simulink model "decoupling_simulation"  (R2018b)
settings: Solver=VariableStepAuto  StartTime=0.0  StopTime=3000  RelTol=1e-3  EnableMultiTasking=on
libraries: simulink x3
settings Model: Creator=38128  LastModifiedBy=99346
settings DataIOCC: LimitDataPoints=on  SaveFormat=Array
settings OptimizationCC: LifeSpan=inf
settings DebuggingCC: SolverPrmCheckMsg=warning  SFUnexpectedBacktrackingDiag=warning  SFNoUnconditionalDefaultTransitionDiag=warning  SFExecutionAtInitializationDiag=none
settings HardwareCC: ProdBitPerPointer=32  ProdBitPerSizeT=32  ProdBitPerPtrDiffT=32  ProdLargestAtomicFloat=None  ProdIntDivRoundTo=Undefined  ProdEndianess=Unspecified  ProdWordSize=32  ProdHWDeviceType=32-bit Generic
settings ModelReferenceCC: PropagateSignalLabelsOutOfModel=off
settings SFSimCC: SimUseLocalCustomCode=off
settings RTWCC: RTWUseLocalCustomCode=off
settings CodeAppCC: StateflowObjectComments=on
settings GRTTargetCC: TargetLangStandard=C89/C90 (ANSI)  GeneratePreprocessorConditionals=Disable all
settings ConfigComp: CovMetricSettings=dw  CovHtmlReporting=on  CovSaveCumulativeToWorkspaceVar=on  CovSaveSingleToWorkspaceVar=on  CovExternalEMLEnable=off  CovSFcnEnable=off

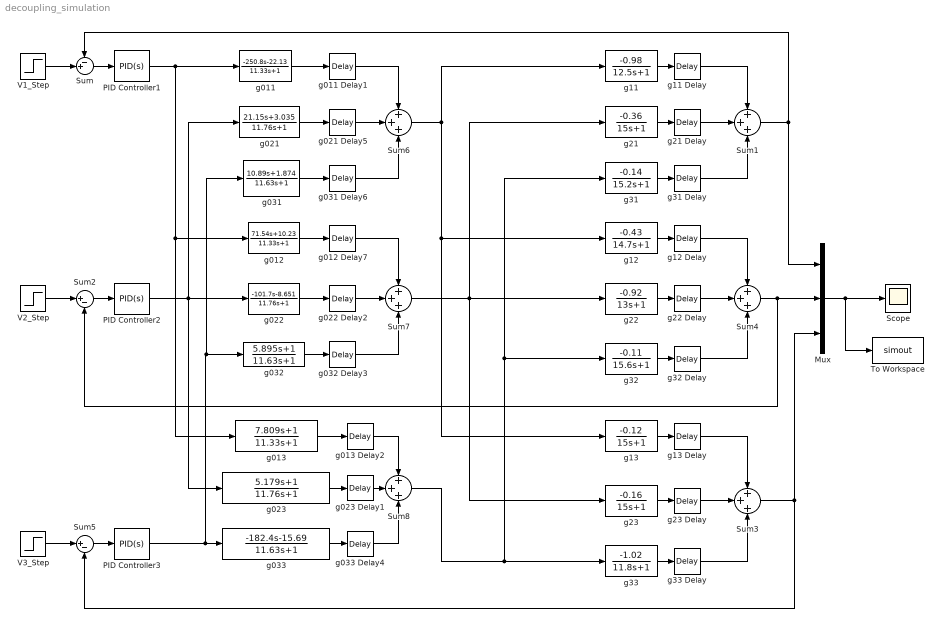
== system decoupling_simulation ==
  Mux : Mux  Inputs=3
  PID Controller1 : simulink/Continuous/PID Controller  Controller=PID  Form=Parallel  TimeDomain=Continuous-time  SampleTime=1  IntegratorMethod=Forward Euler  FilterMethod=Forward Euler  ControllerParametersSource=internal  P=0.0202  I=0.0018  D=0  UseFilter=on  N=100  TunerSelectOption=Transfer Function Based (PID Tuner App)  InitialConditionSource=internal  InitialConditionForIntegrator=0  InitialConditionForFilter=0  DifferentiatorICPrevScaledInput=0  ExternalReset=none  TrackingMode=off  Kt=1  LimitOutput=off  UpperSaturationLimit=inf  LowerSaturationLimit=-inf  LinearizeAsGain=on  AntiWindupMode=none  Kb=1  POutMin=[]  POutMax=[]  IOutMin=[]  IOutMax=[]  DOutMin=[]  DOutMax=[]  NOutMin=[]  NOutMax=[]  SumOutMin=[]  SumOutMax=[]  SaturationOutMin=[]  SaturationOutMax=[]  PParamMin=[]  PParamMax=[]  IParamMin=[]  IParamMax=[]  DParamMin=[]  DParamMax=[]  NParamMin=[]  NParamMax=[]  KbParamMin=[]  KbParamMax=[]  KtParamMin=[]  KtParamMax=[]  KbOutMin=[]  KbOutMax=[]  KtOutMin=[]  KtOutMax=[]  IntegratorOutMin=[]  IntegratorOutMax=[]  FilterOutMin=[]  FilterOutMax=[]  SumI1OutMin=[]  SumI1OutMax=[]  SumI2OutMin=[]  SumI2OutMax=[]  SumI3OutMin=[]  SumI3OutMax=[]  SumI4OutMin=[]  SumI4OutMax=[]  SumDOutMin=[]  SumDOutMax=[]  DifferentiatorOutMin=[]  DifferentiatorOutMax=[]  FilterDiffOutCoefMin=[]  FilterDiffOutCoefMax=[]  ReciprocalOutMin=[]  ReciprocalOutMax=[]  SumDenOutMin=[]  SumDenOutMax=[]  SumNumOutMin=[]  SumNumOutMax=[]  DivideOutMin=[]  DivideOutMax=[]  IntegratorContinuousStateAttributes=''  IntegratorStateMustResolveToSignalObject=off  IntegratorRTWStateStorageClass=Auto  FilterContinuousStateAttributes=''  FilterStateMustResolveToSignalObject=off  FilterRTWStateStorageClass=Auto  ParallelPVariant=InternalParameters  IdealPVariant=Disabled  IVariant=InternalParameters  DVariant=InternalParameters  IntegratorVariant=Continuous  SatVariant=Disabled  AWVariant=Passthrough  PCopyVariant=Disabled  TRVariant=Disabled  FdbkBlocksVariant=Forward  IdealPFdbkVariant=Disabled  SatFdbkVariant=Disabled  DerivativeFilterVariant=ContFilter  NVariant=InternalParameters  NCopyVariant=Disabled  FilterICVariant=InternalICsFilter  IntegratorICVariant=InternalICs  ExternalResetVariant=Disabled  TRSumVariant=Passthrough  SumFdbkVariant=Disabled  SumVariant=Sum_PID
  PID Controller2 : simulink/Continuous/PID Controller  Controller=PID  Form=Parallel  TimeDomain=Continuous-time  SampleTime=1  IntegratorMethod=Forward Euler  FilterMethod=Forward Euler  ControllerParametersSource=internal  P=0.0650  I=0.0055  D=0  UseFilter=on  N=100  TunerSelectOption=Transfer Function Based (PID Tuner App)  InitialConditionSource=internal  InitialConditionForIntegrator=0  InitialConditionForFilter=0  DifferentiatorICPrevScaledInput=0  ExternalReset=none  TrackingMode=off  Kt=1  LimitOutput=off  UpperSaturationLimit=inf  LowerSaturationLimit=-inf  LinearizeAsGain=on  AntiWindupMode=none  Kb=1  POutMin=[]  POutMax=[]  IOutMin=[]  IOutMax=[]  DOutMin=[]  DOutMax=[]  NOutMin=[]  NOutMax=[]  SumOutMin=[]  SumOutMax=[]  SaturationOutMin=[]  SaturationOutMax=[]  PParamMin=[]  PParamMax=[]  IParamMin=[]  IParamMax=[]  DParamMin=[]  DParamMax=[]  NParamMin=[]  NParamMax=[]  KbParamMin=[]  KbParamMax=[]  KtParamMin=[]  KtParamMax=[]  KbOutMin=[]  KbOutMax=[]  KtOutMin=[]  KtOutMax=[]  IntegratorOutMin=[]  IntegratorOutMax=[]  FilterOutMin=[]  FilterOutMax=[]  SumI1OutMin=[]  SumI1OutMax=[]  SumI2OutMin=[]  SumI2OutMax=[]  SumI3OutMin=[]  SumI3OutMax=[]  SumI4OutMin=[]  SumI4OutMax=[]  SumDOutMin=[]  SumDOutMax=[]  DifferentiatorOutMin=[]  DifferentiatorOutMax=[]  FilterDiffOutCoefMin=[]  FilterDiffOutCoefMax=[]  ReciprocalOutMin=[]  ReciprocalOutMax=[]  SumDenOutMin=[]  SumDenOutMax=[]  SumNumOutMin=[]  SumNumOutMax=[]  DivideOutMin=[]  DivideOutMax=[]  IntegratorContinuousStateAttributes=''  IntegratorStateMustResolveToSignalObject=off  IntegratorRTWStateStorageClass=Auto  FilterContinuousStateAttributes=''  FilterStateMustResolveToSignalObject=off  FilterRTWStateStorageClass=Auto  ParallelPVariant=InternalParameters  IdealPVariant=Disabled  IVariant=InternalParameters  DVariant=InternalParameters  IntegratorVariant=Continuous  SatVariant=Disabled  AWVariant=Passthrough  PCopyVariant=Disabled  TRVariant=Disabled  FdbkBlocksVariant=Forward  IdealPFdbkVariant=Disabled  SatFdbkVariant=Disabled  DerivativeFilterVariant=ContFilter  NVariant=InternalParameters  NCopyVariant=Disabled  FilterICVariant=InternalICsFilter  IntegratorICVariant=InternalICs  ExternalResetVariant=Disabled  TRSumVariant=Passthrough  SumFdbkVariant=Disabled  SumVariant=Sum_PID
  PID Controller3 : simulink/Continuous/PID Controller  Controller=PID  Form=Parallel  TimeDomain=Continuous-time  SampleTime=1  IntegratorMethod=Forward Euler  FilterMethod=Forward Euler  ControllerParametersSource=internal  P=0.0247  I=0.0021  D=0  UseFilter=on  N=100  TunerSelectOption=Transfer Function Based (PID Tuner App)  InitialConditionSource=internal  InitialConditionForIntegrator=0  InitialConditionForFilter=0  DifferentiatorICPrevScaledInput=0  ExternalReset=none  TrackingMode=off  Kt=1  LimitOutput=off  UpperSaturationLimit=inf  LowerSaturationLimit=-inf  LinearizeAsGain=on  AntiWindupMode=none  Kb=1  POutMin=[]  POutMax=[]  IOutMin=[]  IOutMax=[]  DOutMin=[]  DOutMax=[]  NOutMin=[]  NOutMax=[]  SumOutMin=[]  SumOutMax=[]  SaturationOutMin=[]  SaturationOutMax=[]  PParamMin=[]  PParamMax=[]  IParamMin=[]  IParamMax=[]  DParamMin=[]  DParamMax=[]  NParamMin=[]  NParamMax=[]  KbParamMin=[]  KbParamMax=[]  KtParamMin=[]  KtParamMax=[]  KbOutMin=[]  KbOutMax=[]  KtOutMin=[]  KtOutMax=[]  IntegratorOutMin=[]  IntegratorOutMax=[]  FilterOutMin=[]  FilterOutMax=[]  SumI1OutMin=[]  SumI1OutMax=[]  SumI2OutMin=[]  SumI2OutMax=[]  SumI3OutMin=[]  SumI3OutMax=[]  SumI4OutMin=[]  SumI4OutMax=[]  SumDOutMin=[]  SumDOutMax=[]  DifferentiatorOutMin=[]  DifferentiatorOutMax=[]  FilterDiffOutCoefMin=[]  FilterDiffOutCoefMax=[]  ReciprocalOutMin=[]  ReciprocalOutMax=[]  SumDenOutMin=[]  SumDenOutMax=[]  SumNumOutMin=[]  SumNumOutMax=[]  DivideOutMin=[]  DivideOutMax=[]  IntegratorContinuousStateAttributes=''  IntegratorStateMustResolveToSignalObject=off  IntegratorRTWStateStorageClass=Auto  FilterContinuousStateAttributes=''  FilterStateMustResolveToSignalObject=off  FilterRTWStateStorageClass=Auto  ParallelPVariant=InternalParameters  IdealPVariant=Disabled  IVariant=InternalParameters  DVariant=InternalParameters  IntegratorVariant=Continuous  SatVariant=Disabled  AWVariant=Passthrough  PCopyVariant=Disabled  TRVariant=Disabled  FdbkBlocksVariant=Forward  IdealPFdbkVariant=Disabled  SatFdbkVariant=Disabled  DerivativeFilterVariant=ContFilter  NVariant=InternalParameters  NCopyVariant=Disabled  FilterICVariant=InternalICsFilter  IntegratorICVariant=InternalICs  ExternalResetVariant=Disabled  TRSumVariant=Passthrough  SumFdbkVariant=Disabled  SumVariant=Sum_PID
  Scope : Scope
  Sum : Sum  Inputs=-+|
  Sum{1,3..4,6..8} (6 alike) : Sum  Inputs=+++
  Sum2 : Sum  Inputs=|+-
  Sum5 : Sum  Inputs=|+-
  To Workspace : ToWorkspace  VariableName=simout  SaveFormat=Timeseries  SampleTime=-1
  V1_Step : Step  Time=2  SampleTime=0
  V2_Step : Step  Time=500  SampleTime=0
  V3_Step : Step  Time=1000  SampleTime=0
  g011 : TransferFcn  Numerator=[-250.8 -22.13]  Denominator=[11.33 1]
  g011 Delay1 : TransportDelay  DelayTime=1.03
  g012 : TransferFcn  Numerator=[71.54 10.23]  Denominator=[11.33 1]
  g012 Delay7 : TransportDelay  DelayTime=3.85
  g013 : TransferFcn  Numerator=[7.809 1]  Denominator=[11.33 1]
  g013 Delay2 : TransportDelay  DelayTime=0
  g021 : TransferFcn  Numerator=[21.15 3.035]  Denominator=[11.76 1]
  g021 Delay5 : TransportDelay  DelayTime=2.62
  g022 : TransferFcn  Numerator=[-101.7 -8.651]  Denominator=[11.76 1]
  g022 Delay2 : TransportDelay  DelayTime=0
  g023 : TransferFcn  Numerator=[5.179 1]  Denominator=[11.76 1]
  g023 Delay1 : TransportDelay  DelayTime=3.52
  g031 : TransferFcn  Numerator=[10.89 1.874]  Denominator=[11.63 1]
  g031 Delay6 : TransportDelay  DelayTime=3.75
  g032 : TransferFcn  Numerator=[5.895 1]  Denominator=[11.63 1]
  g032 Delay3 : TransportDelay  DelayTime=2.4
  g033 : TransferFcn  Numerator=[-182.4 -15.69]  Denominator=[11.63 1]
  g033 Delay4 : TransportDelay  DelayTime=0
  g11 : TransferFcn  Numerator=[-0.98]  Denominator=[12.5 1]
  g11 Delay : TransportDelay  DelayTime=17
  g12 : TransferFcn  Numerator=[-0.43]  Denominator=[14.7 1]
  g12 Delay : TransportDelay  DelayTime=25
  g13 : TransferFcn  Numerator=[-0.12]  Denominator=[15 1]
  g13 Delay : TransportDelay  DelayTime=31
  g21 : TransferFcn  Numerator=[-0.36]  Denominator=[15 1]
  g21 Delay : TransportDelay  DelayTime=27
  g22 : TransferFcn  Numerator=[-0.92]  Denominator=[13 1]
  g22 Delay : TransportDelay  DelayTime=16
  g23 : TransferFcn  Numerator=[-0.16]  Denominator=[15 1]
  g23 Delay : TransportDelay  DelayTime=34
  g31 : TransferFcn  Numerator=[-0.14]  Denominator=[15.2 1]
  g31 Delay : TransportDelay  DelayTime=32
  g32 : TransferFcn  Numerator=[-0.11]  Denominator=[15.6 1]
  g32 Delay : TransportDelay  DelayTime=33
  g33 : TransferFcn  Numerator=[-1.02]  Denominator=[11.8 1]
  g33 Delay : TransportDelay  DelayTime=16
  wires:
  Sum/1 -> PID Controller1/1
  Sum5/1 -> PID Controller3/1
  V1_Step/1 -> Sum/2
  Sum2/1 -> PID Controller2/1
  Mux/1 -> Scope/1, To Workspace/1
  g011/1 -> g011 Delay1/1
  g011 Delay1/1 -> Sum6/1
  PID Controller1/1 -> g011/1, g013/1, g012/1
  g022 Delay2/1 -> Sum7/2
  g032 Delay3/1 -> Sum7/3
  g013 Delay2/1 -> Sum8/1
  g023 Delay1/1 -> Sum8/2
  g033 Delay4/1 -> Sum8/3
  g013/1 -> g013 Delay2/1
  PID Controller2/1 -> g023/1, g022/1, g021/1
  g032/1 -> g032 Delay3/1
  g023/1 -> g023 Delay1/1
  PID Controller3/1 -> g033/1, g032/1, g031/1
  g11/1 -> g11 Delay/1
  g11 Delay/1 -> Sum1/1
  g21/1 -> g21 Delay/1
  g31/1 -> g31 Delay/1
  g21 Delay/1 -> Sum1/2
  g31 Delay/1 -> Sum1/3
  g13/1 -> g13 Delay/1
  g13 Delay/1 -> Sum3/1
  g23/1 -> g23 Delay/1
  g23 Delay/1 -> Sum3/2
  g33 Delay/1 -> Sum3/3
  Sum6/1 -> g11/1, g13/1, g12/1
  Sum7/1 -> g23/1, g22/1, g21/1
  g33/1 -> g33 Delay/1
  Sum8/1 -> g33/1, g32/1, g31/1
  g12/1 -> g12 Delay/1
  g12 Delay/1 -> Sum4/1
  g22/1 -> g22 Delay/1
  g22 Delay/1 -> Sum4/2
  g32 Delay/1 -> Sum4/3
  g32/1 -> g32 Delay/1
  Sum1/1 -> Sum/1, Mux/1
  Sum4/1 -> Mux/2, Sum2/2
  Sum3/1 -> Sum5/2, Mux/3
  V3_Step/1 -> Sum5/1
  V2_Step/1 -> Sum2/1
  g021/1 -> g021 Delay5/1
  g021 Delay5/1 -> Sum6/2
  g031/1 -> g031 Delay6/1
  g031 Delay6/1 -> Sum6/3
  g022/1 -> g022 Delay2/1
  g012/1 -> g012 Delay7/1
  g012 Delay7/1 -> Sum7/1
  g033/1 -> g033 Delay4/1
